simulink model "FlexSensor_Customizable_2in2"  (R2017b)
settings: Solver=VariableStepAuto  StartTime=0.0  StopTime=inf  RelTol=1e-3
libraries: fl_lib x15, nesl_utility x8
settings Model: Creator=stark  LastModifiedBy=stark

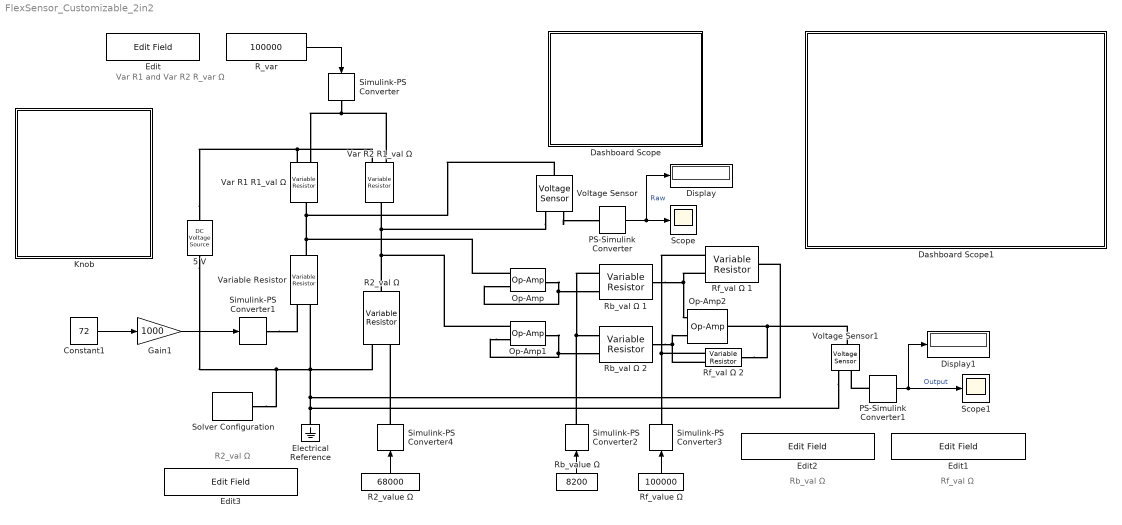
== system FlexSensor_Customizable_2in2 ==
  note: Var R1 and Var R2
      | R_var Ω
  note: Rb_val Ω
  note: Rf_val Ω
  note: R2_val Ω
  5 V : fl_lib/Electrical/Electrical Sources/DC Voltage Source  v0=5 V
  Constant1 : Constant  Value=72
  Dashboard Scope : Subsystem  DialogController=hmiCreateDDGDialog  IsWebBlock=on  mask(MWDashboardBlock){webBlockId=f8f2a28f-58c2-42f2-94c3-86156a7433d8, webBlockType=sdiscope, ShowInitialText=on, HMISrcModelName=FlexSensor_Customizable_2in2}
      mask prompts: webBlockId "WebBlock Id"; webBlockType "WebBlock Type"; HMISrcModelName "Source Model"
      mask help: SimulinkHMI:dialogs:HMIScopeDialogDesc
      mask Help: helpview([docroot '/mapfiles/simulink.map'], 'hmi_scope')
      mask Display:
      | if strcmp(get_param(bdroot(gcb),'BlockDiagramType'), 'library')
      |     image([(matlabroot) '/toolbox/simulink/hmi/icons/DashboardScope.png']);
      | end
  Dashboard Scope1 : Subsystem  DialogController=hmiCreateDDGDialog  IsWebBlock=on  mask(MWDashboardBlock){webBlockId=e5d4e4bc-4844-49fc-94ec-ac60fe534b69, webBlockType=sdiscope, ShowInitialText=on, HMISrcModelName=FlexSensor_Customizable_2in2}
      mask prompts: webBlockId "WebBlock Id"; webBlockType "WebBlock Type"; HMISrcModelName "Source Model"
      mask help: SimulinkHMI:dialogs:HMIScopeDialogDesc
      mask Help: helpview([docroot '/mapfiles/simulink.map'], 'hmi_scope')
      mask Display:
      | if strcmp(get_param(bdroot(gcb),'BlockDiagramType'), 'library')
      |     image([(matlabroot) '/toolbox/simulink/hmi/icons/DashboardScope.png']);
      | end
  Display : Display
  Display1 : Display
  Edit : EditField  WebBlockId=34  ModelName=FlexSensor_Customizable_2in2  LabelPosition=Hide  ShowInitialText=off  Alignment=Center
  Edit1 : EditField  WebBlockId=47  ModelName=FlexSensor_Customizable_2in2  LabelPosition=Hide  ShowInitialText=off  Alignment=Center
  Edit2 : EditField  WebBlockId=48  ModelName=FlexSensor_Customizable_2in2  LabelPosition=Hide  ShowInitialText=off  Alignment=Center
  Edit3 : EditField  WebBlockId=54  ModelName=FlexSensor_Customizable_2in2  LabelPosition=Hide  ShowInitialText=off  Alignment=Center
  Electrical Reference : fl_lib/Electrical/Electrical Elements/Electrical Reference
  Gain1 : Gain  Gain=1000
  Knob : Subsystem  DialogController=hmiCreateDDGDialog  IsWebBlock=on  mask(MWDashboardBlock){webBlockId=99d328bc-3015-47b4-92c2-90252961e884, webBlockType=continuousknob, ShowInLibBrowser=on, ShowInitialText=on, HMISrcModelName=FlexSensor_Customizable_2in2}
      mask prompts: webBlockId "WebBlock Id"; webBlockType "WebBlock Type"; HMISrcModelName "Source Model"
      mask help: SimulinkHMI:dialogs:ContinuousKnobDialogDesc
      mask Help: helpview([docroot '/mapfiles/simulink.map'], 'hmi_knob')
      mask Display:
      | if strcmp(get_param(bdroot(gcb),'BlockDiagramType'), 'library')
      |     image([(matlabroot) '/toolbox/simulink/hmi/icons/ContinuousKnob.png']);
      | end
  Op-Amp : fl_lib/Electrical/Electrical Elements/Op-Amp  outI_specify=off  outI_priority=None  outI=0 A  outI_nominal_specify=off  outI_nominal_unit=A  outI_nominal_value=1
  Op-Amp1 : fl_lib/Electrical/Electrical Elements/Op-Amp  outI_specify=off  outI_priority=None  outI=0 A  outI_nominal_specify=off  outI_nominal_unit=A  outI_nominal_value=1
  Op-Amp2 : fl_lib/Electrical/Electrical Elements/Op-Amp  outI_specify=off  outI_priority=None  outI=0 A  outI_nominal_specify=off  outI_nominal_unit=A  outI_nominal_value=1
  PS-Simulink Converter : nesl_utility/PS-Simulink Converter  PhysicalDomain=network_engine_domain  SubClassName=ps_output  LeftPortType=input  RightPortType=output  PseudoPeriodic=off  Frequencies=[]  Unit=1  AffineConversion=off
  PS-Simulink Converter1 : nesl_utility/PS-Simulink Converter  PhysicalDomain=network_engine_domain  SubClassName=ps_output  LeftPortType=input  RightPortType=output  PseudoPeriodic=off  Frequencies=[]  Unit=1  AffineConversion=off
  R2_val Ω : fl_lib/Electrical/Electrical Elements/Variable Resistor  Rmin=0 Ohm  i_specify=off  i_priority=None  i=0 A  i_nominal_specify=off  i_nominal_unit=A  i_nominal_value=1  v_specify=off  v_priority=None  v=0 V  v_nominal_specify=off  v_nominal_unit=V  v_nominal_value=1
  R2_value Ω : Constant  Value=68000
  R_var : Constant  Value=100000
  Rb_val Ω 1 : fl_lib/Electrical/Electrical Elements/Variable Resistor  Rmin=0 Ohm  i_specify=off  i_priority=None  i=0 A  i_nominal_specify=off  i_nominal_unit=A  i_nominal_value=1  v_specify=off  v_priority=None  v=0 V  v_nominal_specify=off  v_nominal_unit=V  v_nominal_value=1
  Rb_val Ω 2 : fl_lib/Electrical/Electrical Elements/Variable Resistor  Rmin=0 Ohm  i_specify=off  i_priority=None  i=0 A  i_nominal_specify=off  i_nominal_unit=A  i_nominal_value=1  v_specify=off  v_priority=None  v=0 V  v_nominal_specify=off  v_nominal_unit=V  v_nominal_value=1
  Rb_value Ω : Constant  Value=8200
  Rf_val Ω 1 : fl_lib/Electrical/Electrical Elements/Variable Resistor  Rmin=0 Ohm  i_specify=off  i_priority=None  i=0 A  i_nominal_specify=off  i_nominal_unit=A  i_nominal_value=1  v_specify=off  v_priority=None  v=0 V  v_nominal_specify=off  v_nominal_unit=V  v_nominal_value=1
  Rf_val Ω 2 : fl_lib/Electrical/Electrical Elements/Variable Resistor  Rmin=0 Ohm  i_specify=off  i_priority=None  i=0 A  i_nominal_specify=off  i_nominal_unit=A  i_nominal_value=1  v_specify=off  v_priority=None  v=0 V  v_nominal_specify=off  v_nominal_unit=V  v_nominal_value=1
  Rf_value Ω : Constant  Value=100000
  Scope : Scope
  Scope1 : Scope
  Simulink-PS Converter{,1..4} (5 alike) : nesl_utility/Simulink-PS Converter  PhysicalDomain=network_engine_domain  SubClassName=ps_input  LeftPortType=input  RightPortType=output  PseudoPeriodic=off  Frequencies=[]  NoiseDistribution=none  NoiseParameters=[]  Unit=1  AffineConversion=off  FilteringAndDerivatives=provide  SimscapeFilterOrder=1  InputFilterTimeConstant=0.001  UdotUserProvided=0
  Solver Configuration : nesl_utility/Solver Configuration  PhysicalDomain=network_engine_domain  SubClassName=solver  LeftPortType=input  RightPortType=generic  Accelerate=off  Tones=[]  Harmonics=[]  SimulateNoise=off  Profile=off  UseLocalSampling=off  EnableSwitchedLinearOptims=on  FrequencyDomain=off  UseCCode=off  RelTol=0.001  AbsTol=1e-06  MinStep=1e-09  ToWorkspace=off  RevertToSquareIcSolve=off  NumHomotopyIterations=100  PhasorMode=off  PhasorModeNumHarmonics=1  DoDC=off  ResidualTolerance=1e-09  UseLocalSolver=off  LocalSolverChoice=NE_BACKWARD_EULER_ADVANCER  LocalSolverSampleTime=0.001  DoFixedCost=off  MaxNonlinIter=3  MaxModeIter=2  LinearAlgebra=Sparse  DelaysMemoryBudget=1024  AutomaticFiltering=on  FilteringTimeConstant=0.001
  Var R1 R1_val Ω : fl_lib/Electrical/Electrical Elements/Variable Resistor  Rmin=0 Ohm  i_specify=off  i_priority=None  i=0 A  i_nominal_specify=off  i_nominal_unit=A  i_nominal_value=1  v_specify=off  v_priority=None  v=0 V  v_nominal_specify=off  v_nominal_unit=V  v_nominal_value=1
  Var R2 R1_val Ω : fl_lib/Electrical/Electrical Elements/Variable Resistor  Rmin=0 Ohm  i_specify=off  i_priority=None  i=0 A  i_nominal_specify=off  i_nominal_unit=A  i_nominal_value=1  v_specify=off  v_priority=None  v=0 V  v_nominal_specify=off  v_nominal_unit=V  v_nominal_value=1
  Variable Resistor : fl_lib/Electrical/Electrical Elements/Variable Resistor  Rmin=0 Ohm  i_specify=off  i_priority=None  i=0 A  i_nominal_specify=off  i_nominal_unit=A  i_nominal_value=1  v_specify=off  v_priority=None  v=0 V  v_nominal_specify=off  v_nominal_unit=V  v_nominal_value=1
  Voltage Sensor : fl_lib/Electrical/Electrical Sensors/Voltage Sensor
  Voltage Sensor1 : fl_lib/Electrical/Electrical Sensors/Voltage Sensor
  wires:
  Constant1/1 -> Gain1/1
  PS-Simulink Converter/1 -> Display/1, Scope/1  "Raw"
  Gain1/1 -> Simulink-PS Converter1/1
  R_var/1 -> Simulink-PS Converter/1
  PS-Simulink Converter1/1 -> Display1/1, Scope1/1  "Output"
  Rb_value Ω/1 -> Simulink-PS Converter2/1
  Rf_value Ω/1 -> Simulink-PS Converter3/1
  R2_value Ω/1 -> Simulink-PS Converter4/1
  connections:
  Electrical Reference/LConn1 -- Rf_val Ω 1/RConn1 -- Variable Resistor/LConn2 -- R2_val Ω/LConn2 -- 5 V/RConn1 -- Solver Configuration/RConn1 -- Voltage Sensor1/RConn2
  Var R1 R1_val Ω/RConn1 -- Op-Amp/LConn1 -- Variable Resistor/RConn1 -- Voltage Sensor/LConn1
  Op-Amp2/RConn1 -- Rf_val Ω 2/RConn1 -- Voltage Sensor1/LConn1
  Rb_val Ω 2/RConn1 -- Op-Amp2/LConn2 -- Rf_val Ω 2/LConn2
  Var R2 R1_val Ω/RConn1 -- Voltage Sensor/RConn2 -- R2_val Ω/RConn1 -- Op-Amp1/LConn1
  5 V/LConn1 -- Var R1 R1_val Ω/LConn2 -- Var R2 R1_val Ω/LConn2
  Var R2 R1_val Ω/LConn1 -- Simulink-PS Converter/RConn1 -- Var R1 R1_val Ω/LConn1
  Op-Amp/RConn1 -- Op-Amp/LConn2 -- Rb_val Ω 1/LConn2
  Op-Amp1/LConn2 -- Op-Amp1/RConn1 -- Rb_val Ω 2/LConn2
  Rf_val Ω 1/LConn2 -- Op-Amp2/LConn1 -- Rb_val Ω 1/RConn1
  Simulink-PS Converter1/RConn1 -- Variable Resistor/LConn1
  PS-Simulink Converter1/LConn1 -- Voltage Sensor1/RConn1
  Voltage Sensor/RConn1 -- PS-Simulink Converter/LConn1
  Simulink-PS Converter2/RConn1 -- Rb_val Ω 1/LConn1 -- Rb_val Ω 2/LConn1
  Rf_val Ω 2/LConn1 -- Rf_val Ω 1/LConn1 -- Simulink-PS Converter3/RConn1
  Simulink-PS Converter4/RConn1 -- R2_val Ω/LConn1

== system FlexSensor_Customizable_2in2/Dashboard Scope ==

== system FlexSensor_Customizable_2in2/Dashboard Scope1 ==

== system FlexSensor_Customizable_2in2/Knob ==
